simulink model "preamble_header"  (R2025b)
settings: Solver=FixedStepAuto  StartTime=0.0  StopTime=4084  FixedStep=1/1656  RelTol=1e-3
libraries: commsync2 x1
settings Model: VariantFading=off  Creator=karolpalechor  LastModifiedBy=briyi

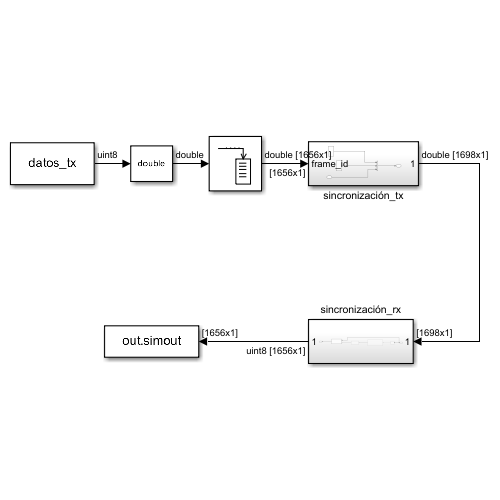
[thumbnail: Simulink's stored preview of the top-level diagram]
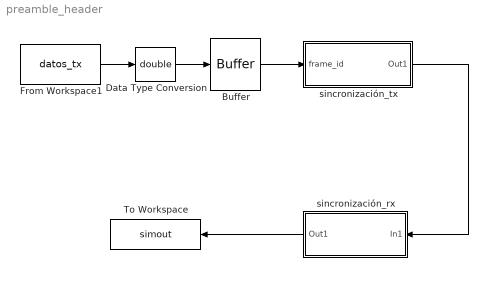
== system preamble_header ==
  Buffer : Buffer  N=1656  OutputFrames=off
  Data Type Conversion : DataTypeConversion  OutDataTypeStr=double  SaturateOnIntegerOverflow=off  RndMeth=Floor
  From Workspace1 : FromWorkspace  VariableName=datos_tx  OutDataTypeStr=uint8  SampleTime=1/1656  Interpolate=off  ZeroCross=off  OutputAfterFinalValue=Holding final value
  To Workspace : ToWorkspace  VariableName=simout  SampleTime=-1
      settings: Save2DSignal=2-D array (concatenate along first dimension)
  sincronización_rx : Subsystem
  sincronización_tx : Subsystem
  wires:
  From Workspace1/1 -> Data Type Conversion/1
  sincronización_tx/1(Out1) -> sincronización_rx/1(In1)
  Data Type Conversion/1 -> Buffer/1
  Buffer/1 -> sincronización_tx/1(frame_id)
  sincronización_rx/1(Out1) -> To Workspace/1

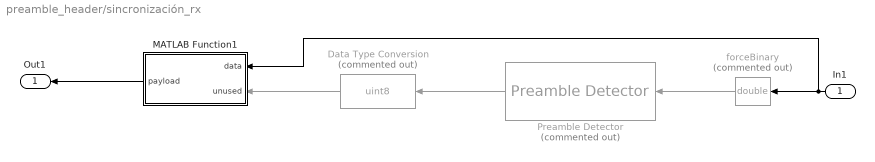
== system preamble_header/sincronización_rx ==
  In1 : Inport
  Data Type Conversion : DataTypeConversion  Commented=on  OutDataTypeStr=uint8  SaturateOnIntegerOverflow=off  RndMeth=Floor
  MATLAB Function1 : MATLAB Function  TreatAsAtomicUnit=on
  Preamble Detector : commsync2/Preamble Detector  Commented=on  Input=Bit  Preamble=[1;1;1;1;1;1;1;1;1;1;0;0;0;0;1;1;1;1;0;0;1;1;0;0;1;1;1;1;1;1;1;1;1;1;0;0;0;0;0;0;0;0]  Threshold=3  DetectionMetricOutput=off  Detections=All  SimulateUsing=Interpreted execution
  forceBinary : DataTypeConversion  Commented=on  OutDataTypeStr=double  SaturateOnIntegerOverflow=off  RndMeth=Floor
  Out1 : Outport
  wires:
  Preamble Detector/1 -> Data Type Conversion/1
  forceBinary/1 -> Preamble Detector/1
  Data Type Conversion/1 -> MATLAB Function1/2(unused)
  MATLAB Function1/1(payload) -> Out1/1
  In1/1 -> forceBinary/1, MATLAB Function1/1(data)

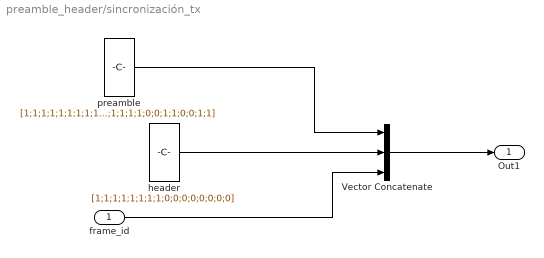
== system preamble_header/sincronización_tx ==
  frame_id : Inport
  Vector Concatenate : Concatenate  NumInputs=3
  header : Constant  Value=[1;1;1;1;1;1;1;1;0;0;0;0;0;0;0;0]  VectorParams1D=off  OutDataTypeStr=double  SampleTime=-1
  preamble : Constant  Value=[1;1;1;1;1;1;1;1;1;1;0;0;0;0;1;1;1;1;0;0;1;1;0;0;1;1]  VectorParams1D=off  OutDataTypeStr=double  SampleTime=-1
  Out1 : Outport
  wires:
  Vector Concatenate/1 -> Out1/1
  preamble/1 -> Vector Concatenate/1
  frame_id/1 -> Vector Concatenate/3
  header/1 -> Vector Concatenate/2

== matlab function preamble_header/sincronización_rx/MATLAB Function1 ==
  data: data input; unused input; payload output
function payload = extract(data, ~)
%#codegen
% Sin canal ruidoso: sync word SIEMPRE en bits 1-42, payload en 43-1698
payload_len = int32(1656);
payload = zeros(payload_len, 1, 'uint8');

for j = int32(1):payload_len
    payload(j) = data(int32(42) + j);
end

end
